simulink model "two_time_domains"  (R2025b)
settings: Solver=ode23tb  StartTime=0.0  StopTime=simlength  MaxStep=tc
undefined symbols (not defined in the file): omega_base, time_gain_afe_module_1, time_gain_afe_module_2, trgo_th_generator, ts_afe
settings Model: Creator=dbagn  LastModifiedBy=dbagn
settings SolverCC: NumberNewtonIterations=3.0  ZeroCrossControl=DisableAll  AlgebraicLoopSolver=TrustRegion  SolverResetMethod=Robust
settings DataIOCC: SaveOutput=off  SignalLogging=off  DSMLogging=off  SaveTime=off  ReturnWorkspaceOutputs=off
settings OptimizationCC: ReuseModelBlockBuffer=off
settings DebuggingCC: UnconnectedInputMsg=warning  UnconnectedOutputMsg=warning  UnconnectedLineMsg=warning
settings ModelReferenceCC: UpdateModelReferenceTargets=Force  EnableRefExpFcnMdlSchedulingChecks=on  ParallelModelReferenceMATLABWorkerInit=Copy Base Workspace
settings SFSimCC: CustomCodeUndefinedFunction=ThrowError  DefaultCustomCodeDeterministicFunctions=All
settings RTWCC: GPUComputeCapability=3.5  DLArmComputeVersion=19.05

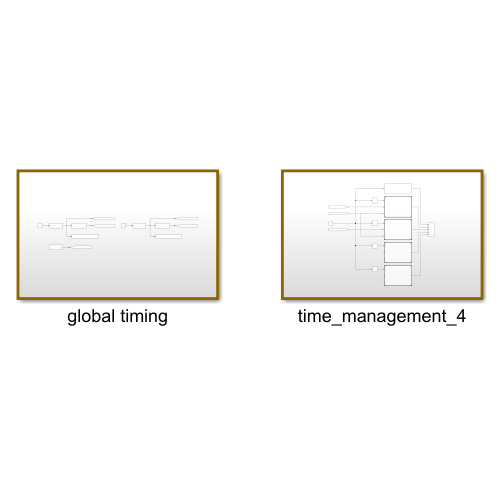
[thumbnail: Simulink's stored preview of the top-level diagram]
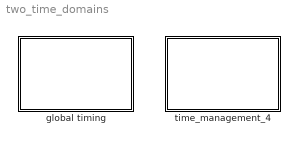
== system two_time_domains ==
  global timing : Subsystem
  time_management_4 : Subsystem

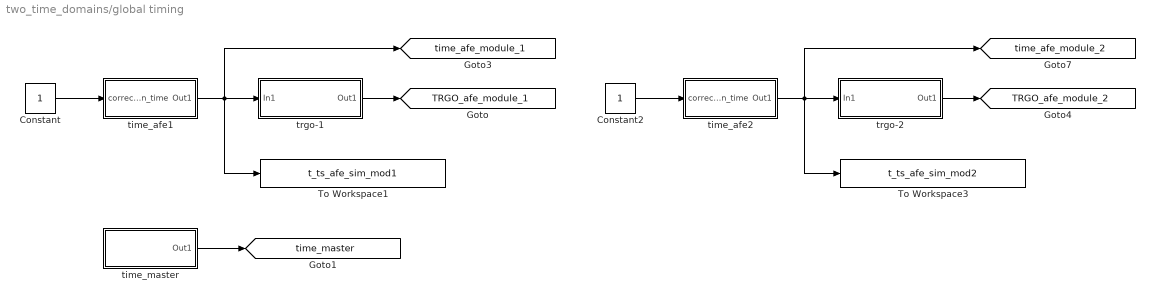
== system two_time_domains/global timing ==
  Constant : Constant
  Constant2 : Constant
  To Workspace1 : ToWorkspace  VariableName=t_ts_afe_sim_mod1  SampleTime=ts_afe
      settings: MaxDataPoints=Ns_afe
  To Workspace3 : ToWorkspace  VariableName=t_ts_afe_sim_mod2  SampleTime=ts_afe
      settings: MaxDataPoints=Ns_afe
  time_afe1 : Subsystem  mask{k=time_gain_afe_module_1}
      mask prompts: k "Time Gain"
      mask Display:
      | disp('time-gen');
      | port_label('input', 1, 'crt');
      | port_label('output', 1, 'tout');
  time_afe2 : Subsystem  mask{k=time_gain_afe_module_2}
      mask prompts: k "Time Gain"
      mask Display:
      | disp('time-gen');
      | port_label('input', 1, 'crt');
      | port_label('output', 1, 'tout');
  time_master : Subsystem  mask{k=1}
      mask prompts: k "Time Gain"
      mask Display:
      | disp('master');
      | port_label('output', 1, 'time');
  trgo-1 : Subsystem  mask{samplig_time=ts_afe}
      mask prompts: samplig_time "Sampling Time"
      mask Display: disp('TRGO Generator');
  trgo-2 : Subsystem  mask{samplig_time=ts_afe}
      mask prompts: samplig_time "Sampling Time"
      mask Display: disp('TRGO Generator');
  tag scope: TRGO_afe_module_1=global, TRGO_afe_module_2=global, time_afe_module_1=global, time_afe_module_2=global, time_master=global
  wires:
  Constant/1 -> time_afe1/1(correction_time)
  time_afe1/1(Out1) -> To Workspace1/1, [time_afe_module_1], trgo-1/1(In1)
  trgo-1/1(Out1) -> [TRGO_afe_module_1]
  trgo-2/1(Out1) -> [TRGO_afe_module_2]
  time_afe2/1(Out1) -> trgo-2/1(In1), [time_afe_module_2], To Workspace3/1
  Constant2/1 -> time_afe2/1(correction_time)
  time_master/1(Out1) -> [time_master]

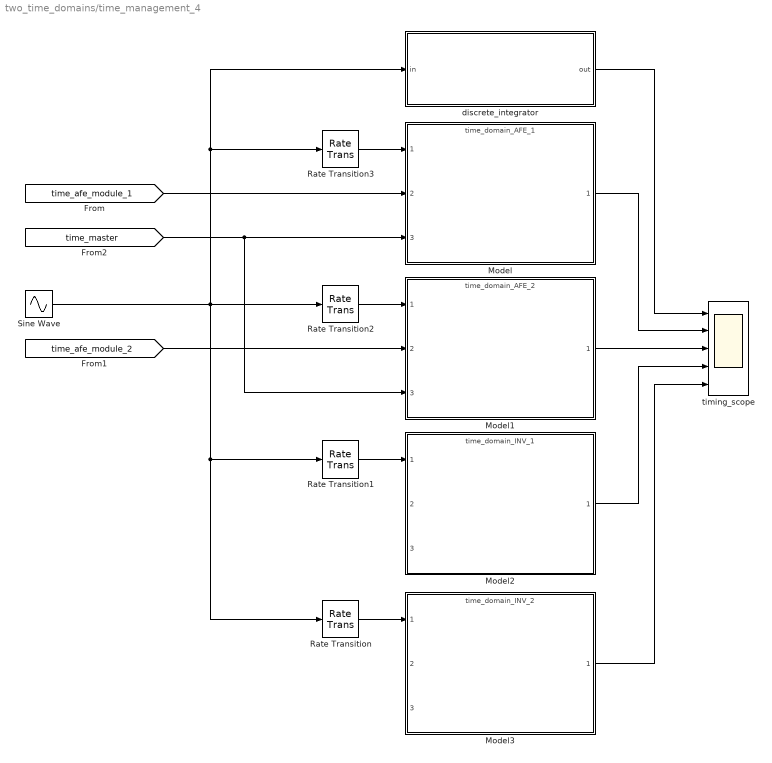
== system two_time_domains/time_management_4 ==
  Model : ModelReference  ModelNameDialog=time_domain_AFE_1  SimulationMode=Normal  ModelReferenceVersion=1.15  CommunicationStepSize=ts_afe_1
  Model1 : ModelReference  ModelNameDialog=time_domain_AFE_2  SimulationMode=Normal  ModelReferenceVersion=1.13  CommunicationStepSize=ts_afe_2
  Model2 : ModelReference  ModelNameDialog=time_domain_INV_1  SimulationMode=Normal  ModelReferenceVersion=1.16  CommunicationStepSize=ts_afe_1
  Model3 : ModelReference  ModelNameDialog=time_domain_INV_2  SimulationMode=Normal  ModelReferenceVersion=1.15  CommunicationStepSize=ts_afe_2
  Rate Transition : RateTransition  OutPortSampleTime=ts_inv_2
  Rate Transition1 : RateTransition  OutPortSampleTime=ts_inv_1
  Rate Transition2 : RateTransition  OutPortSampleTime=ts_afe_2
  Rate Transition3 : RateTransition  OutPortSampleTime=ts_afe_1
  Sine Wave : Sin  Frequency=omega_base  SampleTime=0
  discrete_integrator : Subsystem
  timing_scope : Scope  NumInputPorts=5
      settings: SampleTime=tc  ActiveDisplayYMinimum=1.40096397066399  ActiveDisplayYMaximum=1.74224630212903
  wires:
  Model/1 -> timing_scope/2
  Model1/1 -> timing_scope/3
  discrete_integrator/1(out) -> timing_scope/1
  [time_afe_module_1] -> Model/2
  [time_afe_module_2] -> Model1/2
  [time_master] -> Model1/3, Model/3
  Model2/1 -> timing_scope/4
  Model3/1 -> timing_scope/5
  Sine Wave/1 -> Rate Transition/1, Rate Transition1/1, discrete_integrator/1(in), Rate Transition3/1, Rate Transition2/1
  Rate Transition/1 -> Model3/1
  Rate Transition1/1 -> Model2/1
  Rate Transition2/1 -> Model1/1
  Rate Transition3/1 -> Model/1

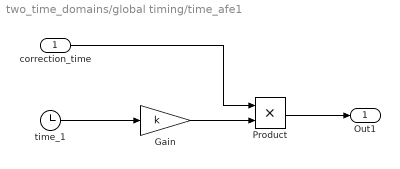
== system two_time_domains/global timing/time_afe1 ==
  correction_time : Inport
  Gain : Gain  Gain=k
  Product : Product
  time_1 : Clock
  Out1 : Outport
  wires:
  time_1/1 -> Gain/1
  Gain/1 -> Product/2
  Product/1 -> Out1/1
  correction_time/1 -> Product/1

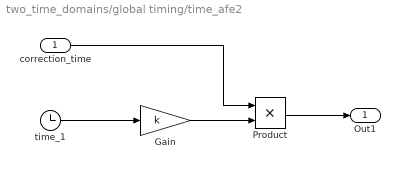
== system two_time_domains/global timing/time_afe2 ==
  correction_time : Inport
  Gain : Gain  Gain=k
  Product : Product
  time_1 : Clock
  Out1 : Outport
  wires:
  correction_time/1 -> Product/1
  Product/1 -> Out1/1
  Gain/1 -> Product/2
  time_1/1 -> Gain/1

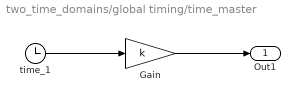
== system two_time_domains/global timing/time_master ==
  Gain : Gain  Gain=k
  time_1 : Clock
  Out1 : Outport
  wires:
  Gain/1 -> Out1/1
  time_1/1 -> Gain/1

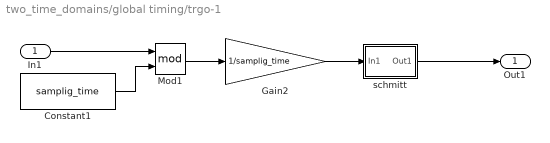
== system two_time_domains/global timing/trgo-1 ==
  In1 : Inport
  Constant1 : Constant  Value=samplig_time
  Gain2 : Gain  Gain=1/samplig_time
  Mod1 : Math  Operator=mod
  schmitt : Subsystem
  Out1 : Outport
  wires:
  Constant1/1 -> Mod1/2
  In1/1 -> Mod1/1
  Mod1/1 -> Gain2/1
  schmitt/1(Out1) -> Out1/1
  Gain2/1 -> schmitt/1(In1)

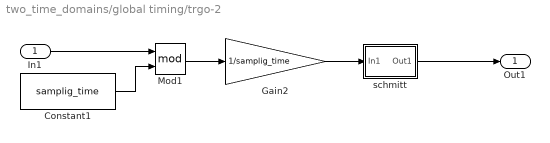
== system two_time_domains/global timing/trgo-2 ==
  In1 : Inport
  Constant1 : Constant  Value=samplig_time
  Gain2 : Gain  Gain=1/samplig_time
  Mod1 : Math  Operator=mod
  schmitt : Subsystem
  Out1 : Outport
  wires:
  Gain2/1 -> schmitt/1(In1)
  schmitt/1(Out1) -> Out1/1
  Mod1/1 -> Gain2/1
  In1/1 -> Mod1/1
  Constant1/1 -> Mod1/2

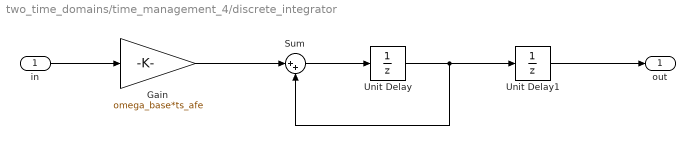
== system two_time_domains/time_management_4/discrete_integrator ==
  in : Inport
  Gain : Gain  Gain=omega_base*ts_afe
  Sum : Sum  Inputs=|++
  Unit Delay : UnitDelay  SampleTime=ts_afe  HasFrameUpgradeWarning=on
  Unit Delay1 : UnitDelay  SampleTime=ts_afe  HasFrameUpgradeWarning=on
  out : Outport
  wires:
  Sum/1 -> Unit Delay/1
  Unit Delay/1 -> Sum/2, Unit Delay1/1
  Gain/1 -> Sum/1
  Unit Delay1/1 -> out/1
  in/1 -> Gain/1

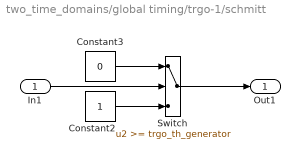
== system two_time_domains/global timing/trgo-1/schmitt ==
  In1 : Inport
  Constant2 : Constant
  Constant3 : Constant  Value=0
  Switch : Switch  Threshold=trgo_th_generator  SaturateOnIntegerOverflow=off  InputSameDT=off
  Out1 : Outport
  wires:
  Constant2/1 -> Switch/3
  Constant3/1 -> Switch/1
  In1/1 -> Switch/2
  Switch/1 -> Out1/1

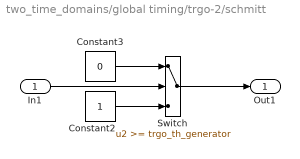
== system two_time_domains/global timing/trgo-2/schmitt ==
  In1 : Inport
  Constant2 : Constant
  Constant3 : Constant  Value=0
  Switch : Switch  Threshold=trgo_th_generator  SaturateOnIntegerOverflow=off  InputSameDT=off
  Out1 : Outport
  wires:
  Switch/1 -> Out1/1
  In1/1 -> Switch/2
  Constant3/1 -> Switch/1
  Constant2/1 -> Switch/3
